simulink model "Simulink block FFT and Inverse Laplace Transform"  (R2025a)
settings: Solver=VariableStepAuto  StartTime=0.0  StopTime=60.5  FixedStep=0.05  RelTol=1e-3
settings Model: Creator=Admin  LastModifiedBy=Admin

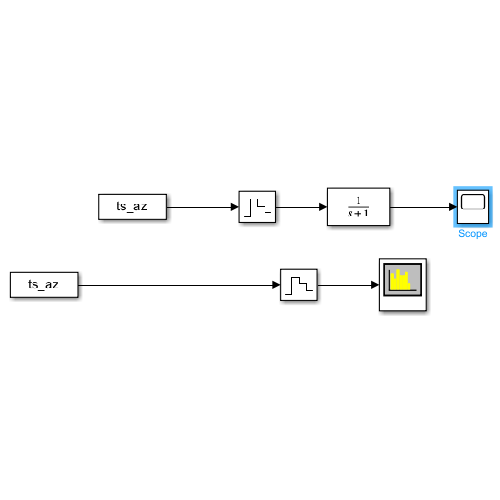
[thumbnail: Simulink's stored preview of the top-level diagram]
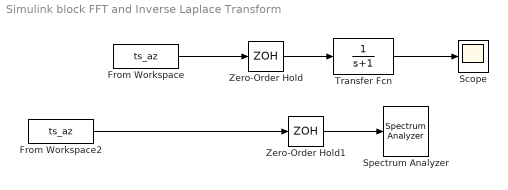
== system Simulink block FFT and Inverse Laplace Transform ==
  From Workspace : FromWorkspace  VariableName=ts_az  SampleTime=0.5
  From Workspace2 : FromWorkspace  VariableName=ts_az  SampleTime=0.5
  Scope : Scope
      settings: ActiveDisplayYMinimum=-0.23759418413535849  ActiveDisplayYMaximum=0.54899091594583993
  Spectrum Analyzer : SpectrumAnalyzer  WindowPosition=[283.000000,134.000000,800.000000,500.000000,]  ScopeFrameLocation=window  SpectrumType=RMS  WindowInvariantSamplesPerUpdate=on  Span=2  StartFrequency=-1  StopFrequency=1  SpectrumUnits=Vrms  YLimits=[-0.0166 0.1505]
  Transfer Fcn : TransferFcn  Denominator=[1 1]
  Zero-Order Hold : ZeroOrderHold  SampleTime=0.5
  Zero-Order Hold1 : ZeroOrderHold  SampleTime=0.5
  wires:
  From Workspace/1 -> Zero-Order Hold/1
  Zero-Order Hold/1 -> Transfer Fcn/1
  Transfer Fcn/1 -> Scope/1
  From Workspace2/1 -> Zero-Order Hold1/1
  Zero-Order Hold1/1 -> Spectrum Analyzer/1
